simulink model "MotionControl"  (R2015b)
settings: Solver=ode3  StartTime=0.0  StopTime=inf  FixedStep=0.05  RelTol=1e-3
undefined symbols (not defined in the file or in its folder): C_nuParams, D, D_nuParams, InitialPos, invM, invT, invThrustAloc, K2, K3, K4, Ki, MAPP1, MAPP2, MAPP3, Sat1Low, Sat1Up, Sat2Low, Sat2Up, Th1, Th2, Th3, Tr, wni, wniCeta2, wnisquared, X, Y, Z
libraries: robotlib x14, realtime_pacer_lib x1
settings Model: Creator=einar  LastModifiedBy=Einar Ueland
settings DataIOCC: ReturnWorkspaceOutputs=on
settings OptimizationCC: OptimizeModelRefInitCode=on  LifeSpan=Inf  MaxStackSize=64
settings DebuggingCC: ReadBeforeWriteMsg=DisableAll  WriteAfterWriteMsg=DisableAll  WriteAfterReadMsg=DisableAll  MultiTaskDSMMsg=none
settings HardwareCC: ProdBitPerPointer=32  ProdLargestAtomicFloat=None  ProdIntDivRoundTo=Undefined  ProdEndianess=Unspecified  ProdWordSize=32  ProdHWDeviceType=Generic->Unspecified (assume 32-bit Generic)
settings ModelReferenceCC: UpdateModelReferenceTargets=IfOutOfDate
settings SFSimCC: SFSimEcho=off
settings RTWCC: SystemTargetFile=ert.tlc  TemplateMakefile=ert_default_tmf  Description=Embedded Coder  Toolchain=Catkin  TargetLang=C++
settings CodeAppCC: IgnoreCustomStorageClasses=off
settings ERTTargetCC: SupportContinuousTime=on

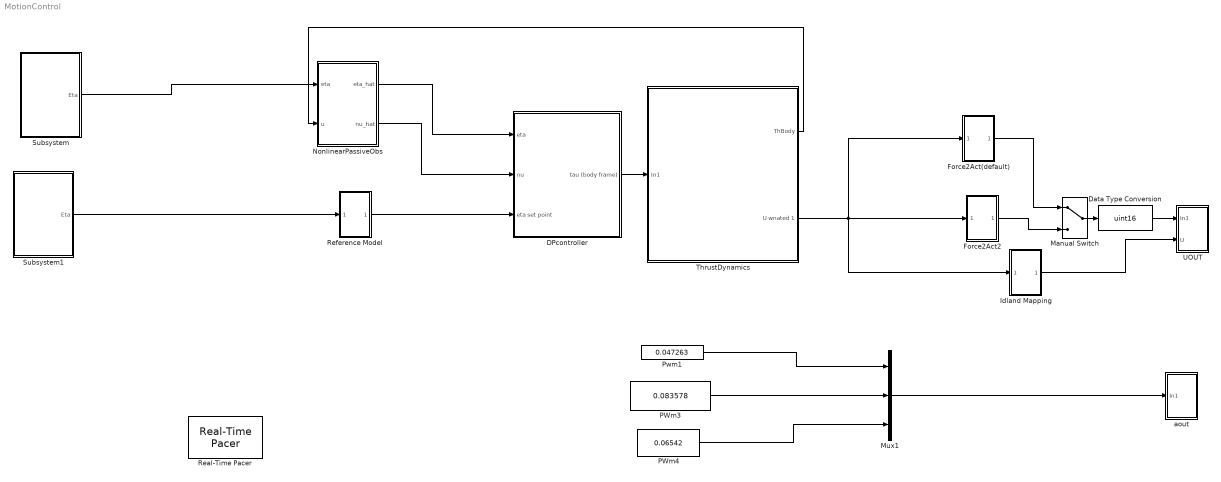
== system MotionControl ==
  DPcontroller : Subsystem
  Data Type Conversion : DataTypeConversion  OutDataTypeStr=uint16
  Force2Act(default) : Subsystem
  Force2Act2 : Subsystem
  Idland Mapping : Subsystem
  Manual Switch : ManualSwitch
  Mux1 : Mux  Inputs=3
  NonlinearPassiveObs : Subsystem
  PWm3 : Constant  Value=0.083578
  PWm4 : Constant  Value=0.06542
  Pwm1 : Constant  Value=0.047263
  Real-Time Pacer : realtime_pacer_lib/Real-Time Pacer  simTimePerRealTime=1
  Reference Model : Subsystem
  Subsystem : Subsystem
  Subsystem1 : Subsystem
  ThrustDynamics : Subsystem
  UOUT : Subsystem
  aout : Subsystem
  wires:
  NonlinearPassiveObs/2(nu_hat) -> DPcontroller/2(nu)
  DPcontroller/1(tau (body frame)) -> ThrustDynamics/1(In1)
  ThrustDynamics/1("ThBody ") -> NonlinearPassiveObs/2(u)
  Reference Model/1(Out1) -> DPcontroller/3(eta set point)
  Subsystem/1(Eta) -> NonlinearPassiveObs/1(eta)
  Subsystem1/1(Eta) -> Reference Model/1(In1)
  Force2Act2/1(Out1) -> Manual Switch/2
  Pwm1/1 -> Mux1/1
  PWm3/1 -> Mux1/2
  PWm4/1 -> Mux1/3
  Mux1/1 -> aout/1(In1)
  NonlinearPassiveObs/1(eta_hat) -> DPcontroller/1(eta)
  ThrustDynamics/2(U wnated 1) -> Force2Act(default)/1(In1), Force2Act2/1(In1), Idland Mapping/1(In1)
  Data Type Conversion/1 -> UOUT/1(In1)
  Idland Mapping/1(Out1) -> UOUT/2(U)
  Manual Switch/1 -> Data Type Conversion/1
  Force2Act(default)/1(Out1) -> Manual Switch/1

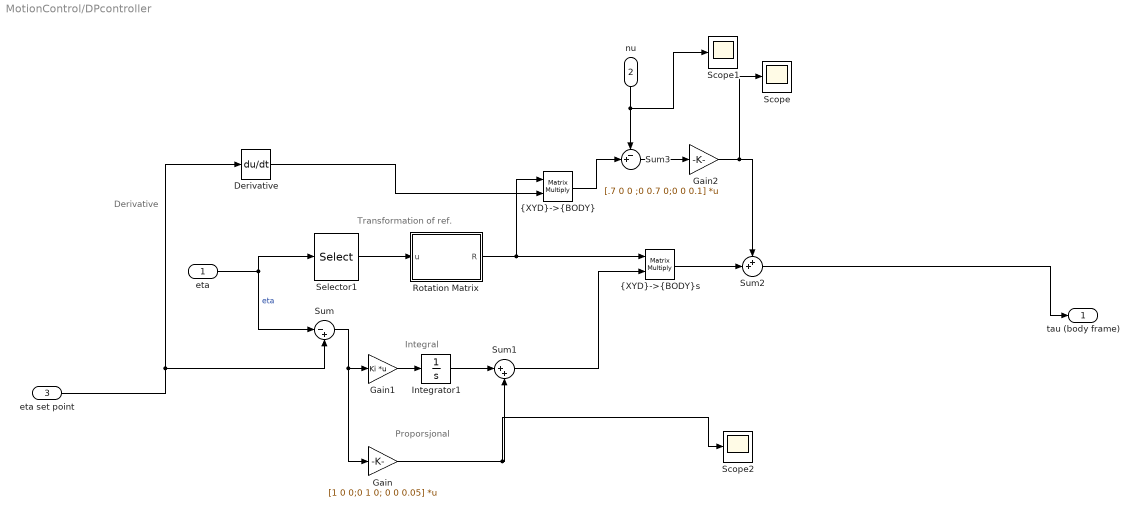
== system MotionControl/DPcontroller ==
  note: Integral
  note: Proporsjonal
  note: Transformation of ref.
  note: Derivative
  eta : Inport
  nu : Inport  Port=2
  eta set point : Inport  Port=3
  Derivative : Derivative
  Gain : Gain  Gain=[1 0 0;0 1 0; 0 0 0.05]  Multiplication=Matrix(K*u)
  Gain1 : Gain  Gain=Ki  Multiplication=Matrix(K*u)
  Gain2 : Gain  Gain=[.7 0 0 ;0 0.7 0;0 0 0.1]  Multiplication=Matrix(K*u)
  Integrator1 : Integrator  InitialCondition=[0;0;0]  LimitOutput=on  UpperSaturationLimit=[1;1;1]  LowerSaturationLimit=[-1;-1;-1]
  Rotation Matrix : MATLAB Function  TreatAsAtomicUnit=on
  Scope : Scope
  Scope1 : Scope
  Scope2 : Scope
  Selector1 : Selector  InputPortWidth=3  IndexOptions=Index vector (dialog)  Indices=[3]  OutputSizes=1
  Sum : Sum  Inputs=|-+
  Sum1 : Sum  Inputs=|++
  Sum2 : Sum  Inputs=++|
  Sum3 : Sum  Inputs=-+|
  "{XYD}->{BODY}" : Product  Multiplication=Matrix(*)
  "{XYD}->{BODY}s" : Product  Multiplication=Matrix(*)
  tau (body frame) : Outport
  wires:
  eta/1 -> Selector1/1, Sum/1  "eta"
  Sum/1 -> Gain1/1, Gain/1
  Selector1/1 -> Rotation Matrix/1(u)
  Rotation Matrix/1(R) -> "{XYD}->{BODY}"/1, "{XYD}->{BODY}s"/1
  Sum2/1 -> tau (body frame)/1
  Gain1/1 -> Integrator1/1
  Gain/1 -> Scope2/1, Sum1/2
  Sum1/1 -> "{XYD}->{BODY}s"/2
  Derivative/1 -> "{XYD}->{BODY}"/2
  "{XYD}->{BODY}s"/1 -> Sum2/2
  nu/1 -> Scope1/1, Sum3/1
  "{XYD}->{BODY}"/1 -> Sum3/2
  Sum3/1 -> Gain2/1
  Gain2/1 -> Scope/1, Sum2/1
  eta set point/1 -> Sum/2, Derivative/1
  Integrator1/1 -> Sum1/1

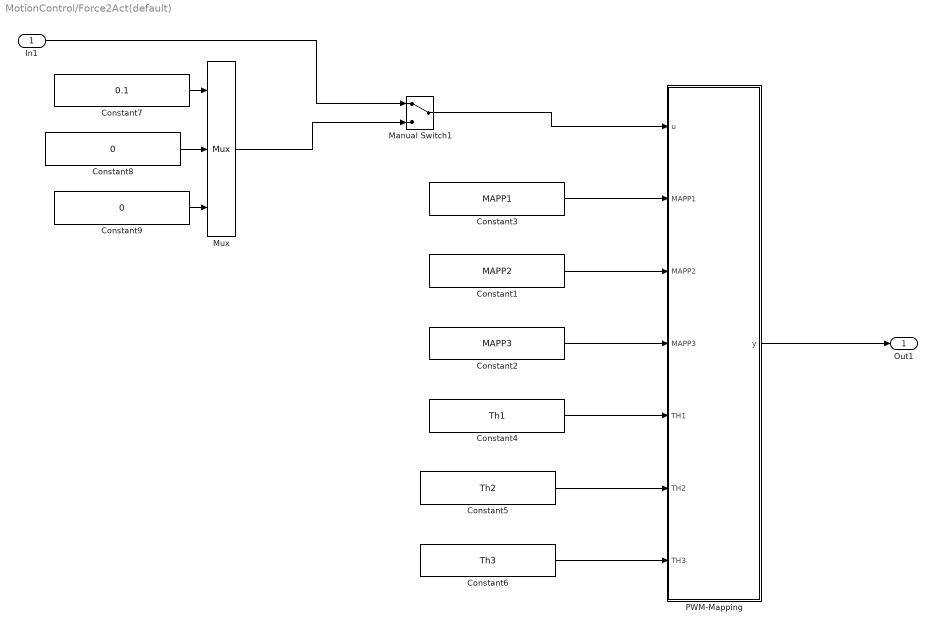
== system MotionControl/Force2Act(default) ==
  In1 : Inport
  Constant1 : Constant  Value=MAPP2
  Constant2 : Constant  Value=MAPP3
  Constant3 : Constant  Value=MAPP1
  Constant4 : Constant  Value=Th1
  Constant5 : Constant  Value=Th2
  Constant6 : Constant  Value=Th3
  Constant7 : Constant  Value=0.1
  Constant8 : Constant  Value=0
  Constant9 : Constant  Value=0
  Manual Switch1 : ManualSwitch
  Mux : Mux  Inputs=3
  PWM-Mapping : MATLAB Function  TreatAsAtomicUnit=on
  Out1 : Outport
  wires:
  Manual Switch1/1 -> PWM-Mapping/1(u)
  Constant4/1 -> PWM-Mapping/5(TH1)
  Constant6/1 -> PWM-Mapping/7(TH3)
  Constant5/1 -> PWM-Mapping/6(TH2)
  Constant3/1 -> PWM-Mapping/2(MAPP1)
  Constant1/1 -> PWM-Mapping/3(MAPP2)
  Constant2/1 -> PWM-Mapping/4(MAPP3)
  PWM-Mapping/1(y) -> Out1/1
  In1/1 -> Manual Switch1/1
  Constant7/1 -> Mux/1
  Constant8/1 -> Mux/2
  Mux/1 -> Manual Switch1/2
  Constant9/1 -> Mux/3

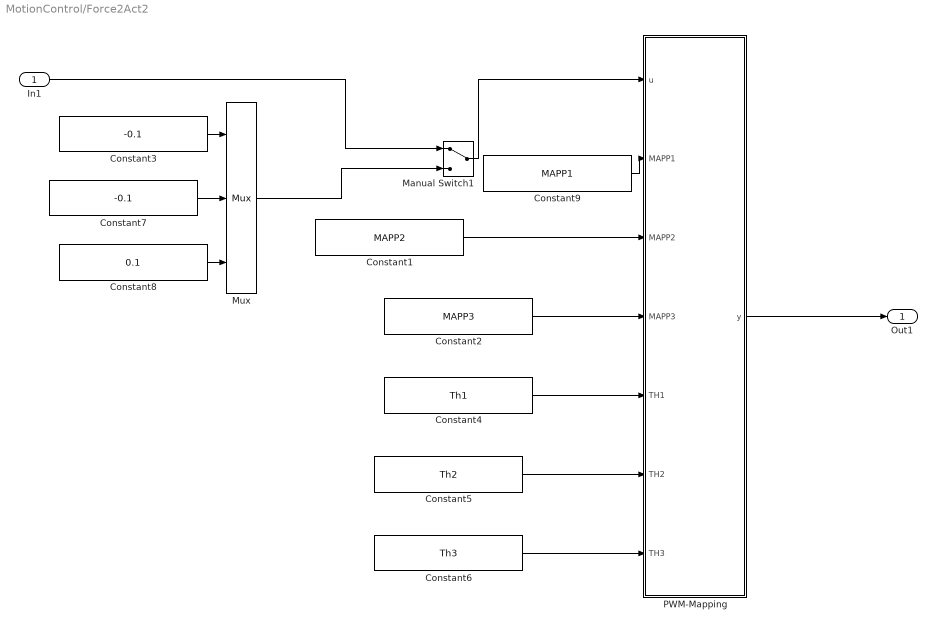
== system MotionControl/Force2Act2 ==
  In1 : Inport
  Constant1 : Constant  Value=MAPP2
  Constant2 : Constant  Value=MAPP3
  Constant3 : Constant  Value=-0.1
  Constant4 : Constant  Value=Th1
  Constant5 : Constant  Value=Th2
  Constant6 : Constant  Value=Th3
  Constant7 : Constant  Value=-0.1
  Constant8 : Constant  Value=0.1
  Constant9 : Constant  Value=MAPP1
  Manual Switch1 : ManualSwitch
  Mux : Mux  Inputs=3
  PWM-Mapping : MATLAB Function  TreatAsAtomicUnit=on
  Out1 : Outport
  wires:
  PWM-Mapping/1(y) -> Out1/1
  Constant2/1 -> PWM-Mapping/4(MAPP3)
  Constant1/1 -> PWM-Mapping/3(MAPP2)
  Manual Switch1/1 -> PWM-Mapping/1(u)
  Constant5/1 -> PWM-Mapping/6(TH2)
  Constant6/1 -> PWM-Mapping/7(TH3)
  Constant4/1 -> PWM-Mapping/5(TH1)
  In1/1 -> Manual Switch1/1
  Constant8/1 -> Mux/3
  Constant3/1 -> Mux/1
  Constant7/1 -> Mux/2
  Mux/1 -> Manual Switch1/2
  Constant9/1 -> PWM-Mapping/2(MAPP1)

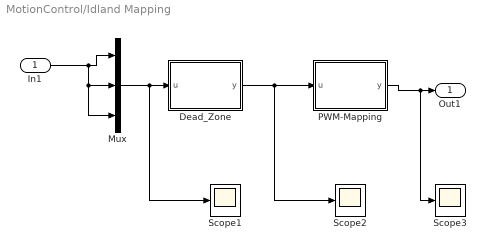
== system MotionControl/Idland Mapping ==
  In1 : Inport
  Dead_Zone : MATLAB Function  TreatAsAtomicUnit=on
  Mux : Mux  Inputs=3
  PWM-Mapping : MATLAB Function  TreatAsAtomicUnit=on
  Scope1 : Scope
  Scope2 : Scope
  Scope3 : Scope
  Out1 : Outport
  wires:
  PWM-Mapping/1(y) -> Out1/1, Scope3/1
  Mux/1 -> Dead_Zone/1(u), Scope1/1
  In1/1 -> Mux/3, Mux/2, Mux/1
  Dead_Zone/1(y) -> PWM-Mapping/1(u), Scope2/1

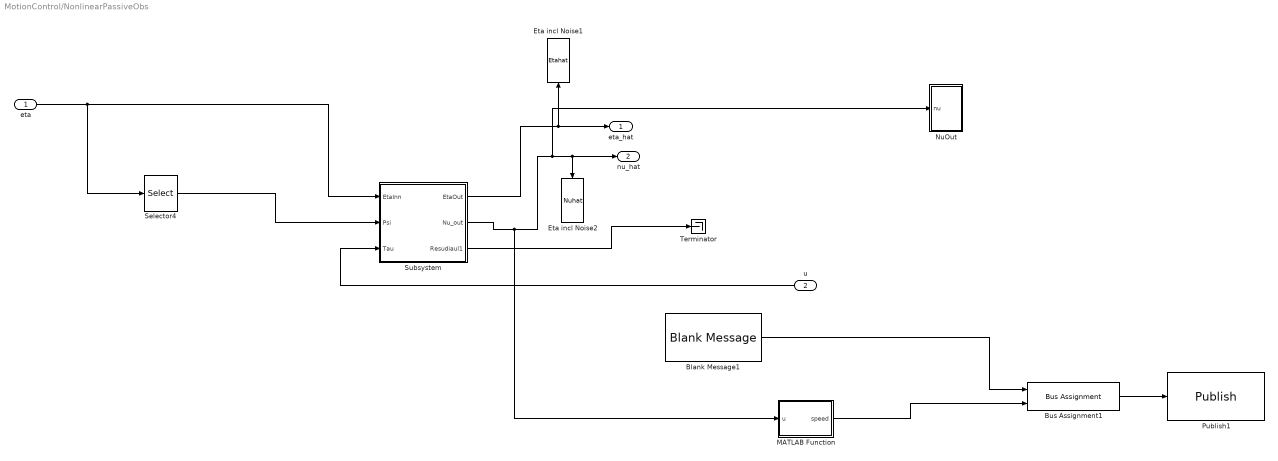
== system MotionControl/NonlinearPassiveObs ==
  eta : Inport
  u : Inport  Port=2
  Blank Message1 : robotlib/Blank Message  SourceLibraryInfo=This block requires Robotics System Toolbox  messageType=std_msgs/Float64  SampleTime=inf
  Bus Assignment1 : BusAssignment  AssignedSignals=Data
  Eta incl Noise1 : ToWorkspace  VariableName=Etahat  SaveFormat=Timeseries  SampleTime=-1
  Eta incl Noise2 : ToWorkspace  VariableName=Nuhat  SaveFormat=Timeseries  SampleTime=-1
  MATLAB Function : MATLAB Function  TreatAsAtomicUnit=on
  NuOut : Subsystem
  Publish1 : robotlib/Publish  SourceLibraryInfo=This block requires Robotics System Toolbox  topicSource=Specify your own  topic=/VesselSpeed  messageType=std_msgs/Float64  messageQueueLength=1
  Selector4 : Selector  InputPortWidth=3  IndexOptions=Index vector (dialog)  Indices=3  OutputSizes=1
  Subsystem : Subsystem
  Terminator : Terminator
  eta_hat : Outport
  nu_hat : Outport  Port=2
  wires:
  Subsystem/3("Resudiaul1 ") -> Terminator/1
  eta/1 -> Selector4/1, Subsystem/1(EtaInn)
  Selector4/1 -> Subsystem/2(Psi)
  u/1 -> Subsystem/3("Tau ")
  Subsystem/1("EtaOut ") -> Eta incl Noise1/1, eta_hat/1
  Bus Assignment1/1 -> Publish1/1
  Blank Message1/1 -> Bus Assignment1/1
  Subsystem/2("Nu_out ") -> MATLAB Function/1(u), NuOut/1("nu "), Eta incl Noise2/1, nu_hat/1
  MATLAB Function/1(speed) -> Bus Assignment1/2

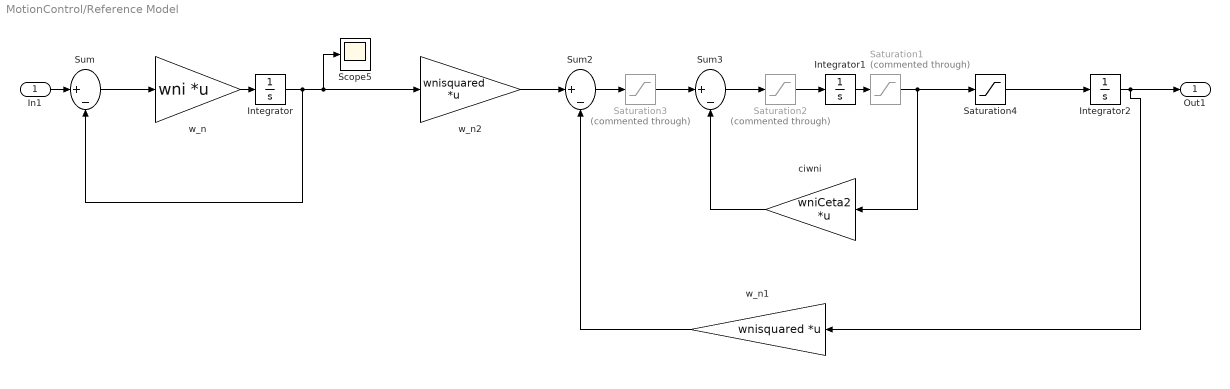
== system MotionControl/Reference Model ==
  In1 : Inport
  Integrator : Integrator  InitialCondition=[0;0;0]
  Integrator1 : Integrator  InitialCondition=[0 ;0; 0]
  Integrator2 : Integrator  InitialCondition=[0;0;0]
  Saturation1 : Saturate  Commented=through  UpperLimit=Sat2Up  LowerLimit=Sat2Low
  Saturation2 : Saturate  Commented=through  UpperLimit=Sat1Up  LowerLimit=Sat1Low
  Saturation3 : Saturate  Commented=through  UpperLimit=Sat1Up  LowerLimit=Sat1Low
  Saturation4 : Saturate  UpperLimit=Sat2Up  LowerLimit=Sat2Low
  Scope5 : Scope
  Sum : Sum  Inputs=|+-
  Sum2 : Sum  Inputs=|+-
  Sum3 : Sum  Inputs=|+-
  ciwni : Gain  Gain=wniCeta2  Multiplication=Matrix(K*u)
  w_n : Gain  Gain=wni  Multiplication=Matrix(K*u)
  w_n1 : Gain  Gain=wnisquared  Multiplication=Matrix(K*u)
  w_n2 : Gain  Gain=wnisquared  Multiplication=Matrix(K*u)
  Out1 : Outport
  wires:
  w_n/1 -> Integrator/1
  w_n2/1 -> Sum2/1
  Integrator/1 -> Scope5/1, w_n2/1, Sum/2
  Integrator2/1 -> Out1/1, w_n1/1
  ciwni/1 -> Sum3/2
  Saturation1/1 -> ciwni/1, Saturation4/1
  Saturation2/1 -> Integrator1/1
  Sum2/1 -> Saturation3/1
  Sum3/1 -> Saturation2/1
  Sum/1 -> w_n/1
  In1/1 -> Sum/1
  Integrator1/1 -> Saturation1/1
  w_n1/1 -> Sum2/2
  Saturation3/1 -> Sum3/1
  Saturation4/1 -> Integrator2/1

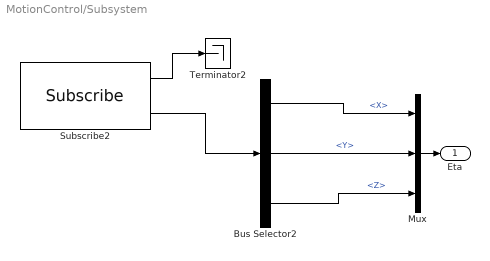
== system MotionControl/Subsystem ==
  Bus Selector2 : BusSelector  OutputSignals=X,Y,Z
  Mux : Mux  Inputs=3
  Subscribe2 : robotlib/Subscribe  SourceLibraryInfo=This block requires Robotics System Toolbox  topicSource=Specify your own  topic=/Eta  messageType=geometry_msgs/Vector3  sampleTime=-1  messageQueueLength=1
  Terminator2 : Terminator
  Eta : Outport
  wires:
  Bus Selector2/1 -> Mux/1  "<X>"
  Subscribe2/2 -> Bus Selector2/1
  Mux/1 -> Eta/1
  Subscribe2/1 -> Terminator2/1
  Bus Selector2/2 -> Mux/2  "<Y>"
  Bus Selector2/3 -> Mux/3  "<Z>"

== system MotionControl/Subsystem1 ==
  Bus Selector2 : BusSelector  OutputSignals=X,Y,Z
  Mux : Mux  Inputs=3
  Subscribe2 : robotlib/Subscribe  SourceLibraryInfo=This block requires Robotics System Toolbox  topicSource=Specify your own  topic=/Position  messageType=geometry_msgs/Vector3  sampleTime=-1  messageQueueLength=1
  Terminator2 : Terminator
  Eta : Outport
  wires:
  Subscribe2/2 -> Bus Selector2/1
  Mux/1 -> Eta/1
  Subscribe2/1 -> Terminator2/1
  Bus Selector2/1 -> Mux/1  "<X>"
  Bus Selector2/2 -> Mux/2  "<Y>"
  Bus Selector2/3 -> Mux/3  "<Z>"

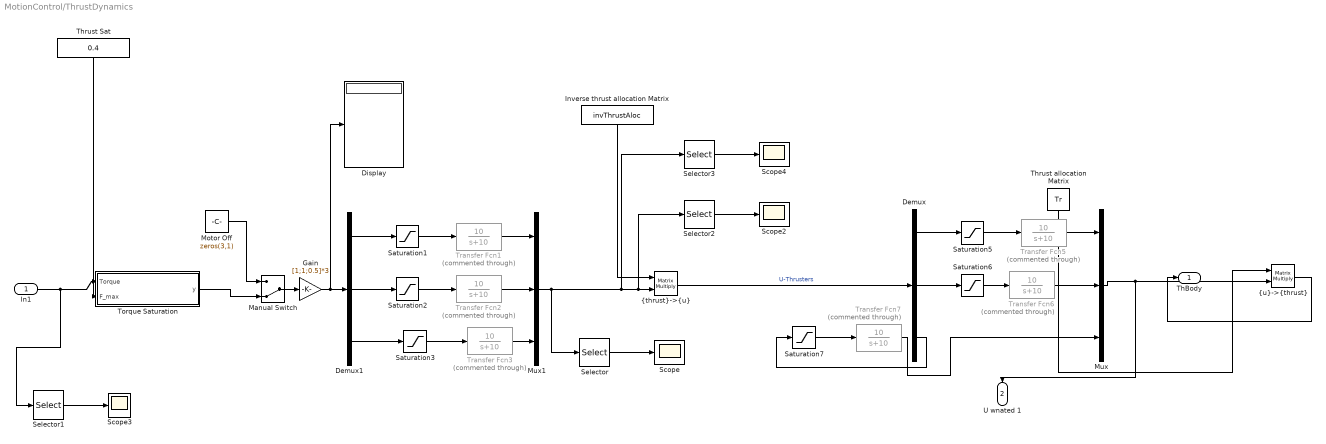
== system MotionControl/ThrustDynamics ==
  In1 : Inport
  Demux : Demux  Outputs=3
  Demux1 : Demux  Outputs=3
  Display : Display
  Gain : Gain  Gain=[1;1;0.5]*3
  Inverse thrust allocation Matrix : Constant  Value=invThrustAloc
  Manual Switch : ManualSwitch  CurrentSetting=0
  Motor Off : Constant  Value=zeros(3,1)
  Mux : Mux  Inputs=3
  Mux1 : Mux  Inputs=3
  Saturation1 : Saturate  UpperLimit=1  LowerLimit=-1  ZeroCross=off
  Saturation2 : Saturate  UpperLimit=1  LowerLimit=-1  ZeroCross=off
  Saturation3 : Saturate  UpperLimit=0.05  LowerLimit=-0.05  ZeroCross=off
  Saturation5 : Saturate  UpperLimit=4  LowerLimit=-4  ZeroCross=off
  Saturation6 : Saturate  UpperLimit=4  LowerLimit=-4  ZeroCross=off
  Saturation7 : Saturate  UpperLimit=4  LowerLimit=-4  ZeroCross=off
  Scope{,2..4} (4 alike) : Scope
  Selector : Selector  InputPortWidth=3  IndexOptions=Index vector (dialog)  Indices=[3]  OutputSizes=1
  Selector1 : Selector  InputPortWidth=3  IndexOptions=Index vector (dialog)  Indices=[3]  OutputSizes=1
  Selector2 : Selector  InputPortWidth=3  IndexOptions=Index vector (dialog)  Indices=2  OutputSizes=1
  Selector3 : Selector  InputPortWidth=3  IndexOptions=Index vector (dialog)  Indices=1  OutputSizes=1
  Thrust Sat : Constant  Value=0.4
  Thrust allocation Matrix : Constant  Value=Tr
  Torque Saturation : MATLAB Function  TreatAsAtomicUnit=on
  Transfer Fcn{1..3,5..7} (6 alike) : TransferFcn  Commented=through  Numerator=[10]  Denominator=[1 10]
  "{thrust}->{u}" : Product  Multiplication=Matrix(*)
  "{u}->{thrust}" : Product  Multiplication=Matrix(*)
  "ThBody " : Outport
  U wnated 1 : Outport  Port=2
  wires:
  Demux/1 -> Saturation5/1
  Demux/2 -> Saturation6/1
  Demux/3 -> Saturation7/1
  "{u}->{thrust}"/1 -> "ThBody "/1
  Thrust allocation Matrix/1 -> "{u}->{thrust}"/1
  Mux/1 -> "{u}->{thrust}"/2, U wnated 1/1
  "{thrust}->{u}"/1 -> Demux/1  "U-Thrusters"
  Inverse thrust allocation Matrix/1 -> "{thrust}->{u}"/1
  Saturation7/1 -> Transfer Fcn7/1
  Saturation6/1 -> Transfer Fcn6/1
  Saturation5/1 -> Transfer Fcn5/1
  Transfer Fcn5/1 -> Mux/1
  Transfer Fcn7/1 -> Mux/3
  Transfer Fcn6/1 -> Mux/2
  Selector/1 -> Scope/1
  In1/1 -> Selector1/1, Torque Saturation/1(Torque)
  Selector1/1 -> Scope3/1
  Demux1/1 -> Saturation1/1
  Demux1/2 -> Saturation2/1
  Demux1/3 -> Saturation3/1
  Saturation3/1 -> Transfer Fcn3/1
  Saturation2/1 -> Transfer Fcn2/1
  Saturation1/1 -> Transfer Fcn1/1
  Transfer Fcn1/1 -> Mux1/1
  Transfer Fcn3/1 -> Mux1/3
  Transfer Fcn2/1 -> Mux1/2
  Gain/1 -> Display/1, Demux1/1
  Mux1/1 -> Selector/1, Selector3/1, Selector2/1, "{thrust}->{u}"/2
  Selector2/1 -> Scope2/1
  Selector3/1 -> Scope4/1
  Thrust Sat/1 -> Torque Saturation/2(F_max)
  Torque Saturation/1(y) -> Manual Switch/2
  Manual Switch/1 -> Gain/1
  Motor Off/1 -> Manual Switch/1

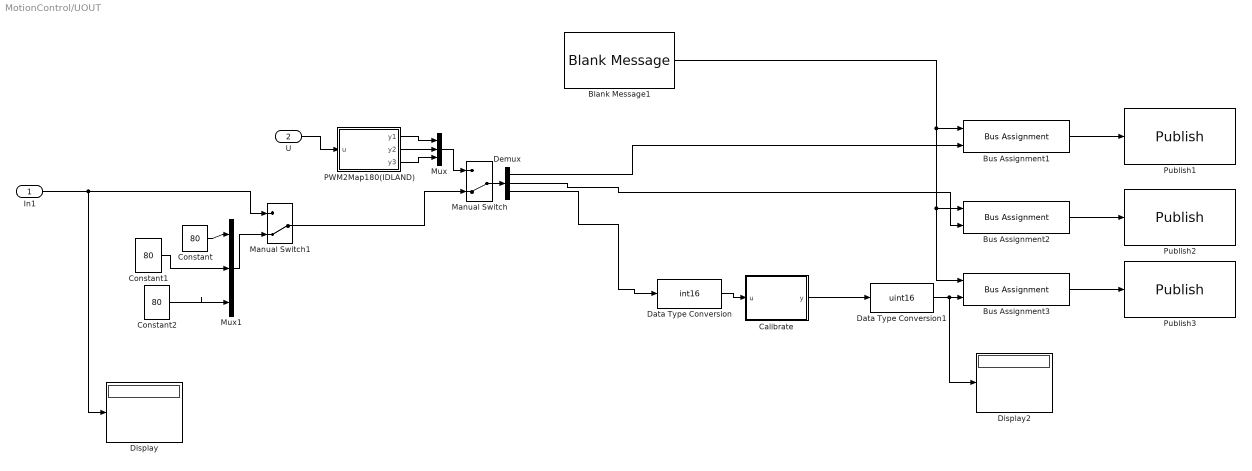
== system MotionControl/UOUT ==
  In1 : Inport
  U : Inport  Port=2
  Blank Message1 : robotlib/Blank Message  SourceLibraryInfo=This block requires Robotics System Toolbox  messageType=std_msgs/UInt16  SampleTime=inf
  Bus Assignment1 : BusAssignment  AssignedSignals=Data
  Bus Assignment2 : BusAssignment  AssignedSignals=Data
  Bus Assignment3 : BusAssignment  AssignedSignals=Data
  Calibrate : MATLAB Function  TreatAsAtomicUnit=on
  Constant : Constant  Value=80  OutDataTypeStr=uint16
  Constant1 : Constant  Value=80  OutDataTypeStr=uint16
  Constant2 : Constant  Value=80  OutDataTypeStr=uint16
  Data Type Conversion : DataTypeConversion  OutDataTypeStr=int16
  Data Type Conversion1 : DataTypeConversion  OutDataTypeStr=uint16
  Demux : Demux  Outputs=3
  Display : Display
  Display2 : Display
  Manual Switch : ManualSwitch  CurrentSetting=0
  Manual Switch1 : ManualSwitch  CurrentSetting=0
  Mux : Mux  Inputs=3
  Mux1 : Mux  Inputs=3
  "PWM2Map180(IDLAND) " : MATLAB Function  TreatAsAtomicUnit=on
  Publish1 : robotlib/Publish  SourceLibraryInfo=This block requires Robotics System Toolbox  topicSource=Specify your own  topic=/Thrust1  messageType=std_msgs/UInt16  messageQueueLength=1
  Publish2 : robotlib/Publish  SourceLibraryInfo=This block requires Robotics System Toolbox  topicSource=Specify your own  topic=/Thrust2  messageType=std_msgs/UInt16  messageQueueLength=1
  Publish3 : robotlib/Publish  SourceLibraryInfo=This block requires Robotics System Toolbox  topicSource=Specify your own  topic=/Thrust3  messageType=std_msgs/UInt16  messageQueueLength=1
  wires:
  Bus Assignment3/1 -> Publish3/1
  Demux/2 -> Bus Assignment2/2
  Bus Assignment1/1 -> Publish1/1
  Blank Message1/1 -> Bus Assignment3/1, Bus Assignment2/1, Bus Assignment1/1
  In1/1 -> Manual Switch1/1, Display/1
  Demux/1 -> Bus Assignment1/2
  Bus Assignment2/1 -> Publish2/1
  U/1 -> "PWM2Map180(IDLAND) "/1(u)
  "PWM2Map180(IDLAND) "/2(y2) -> Mux/2
  "PWM2Map180(IDLAND) "/3(y3) -> Mux/3
  "PWM2Map180(IDLAND) "/1(y1) -> Mux/1
  Mux/1 -> Manual Switch/1
  Manual Switch/1 -> Demux/1
  Mux1/1 -> Manual Switch1/2
  Constant/1 -> Mux1/1
  Constant1/1 -> Mux1/2
  Constant2/1 -> Mux1/3
  Manual Switch1/1 -> Manual Switch/2
  Demux/3 -> Data Type Conversion/1
  Data Type Conversion/1 -> Calibrate/1(u)
  Data Type Conversion1/1 -> Display2/1, Bus Assignment3/2
  Calibrate/1(y) -> Data Type Conversion1/1

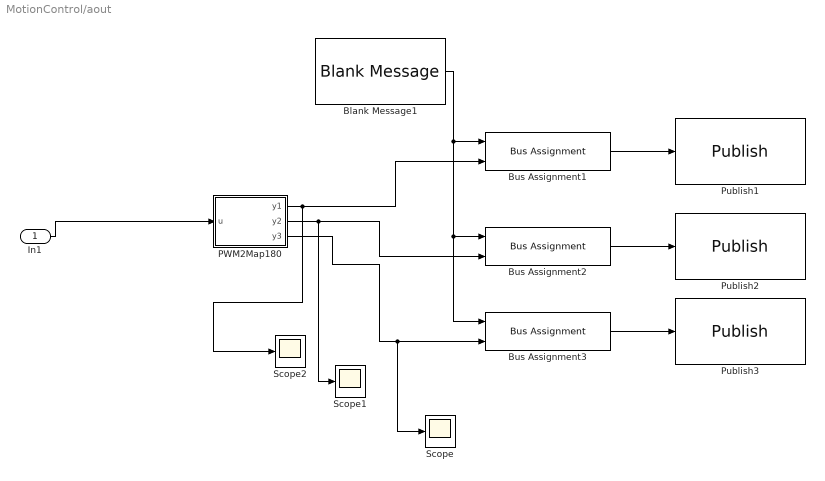
== system MotionControl/aout ==
  In1 : Inport
  Blank Message1 : robotlib/Blank Message  SourceLibraryInfo=This block requires Robotics System Toolbox  messageType=std_msgs/UInt16  SampleTime=inf
  Bus Assignment1 : BusAssignment  AssignedSignals=Data
  Bus Assignment2 : BusAssignment  AssignedSignals=Data
  Bus Assignment3 : BusAssignment  AssignedSignals=Data
  "PWM2Map180 " : MATLAB Function  TreatAsAtomicUnit=on
  Publish1 : robotlib/Publish  SourceLibraryInfo=This block requires Robotics System Toolbox  topicSource=Specify your own  topic=/a1  messageType=std_msgs/UInt16  messageQueueLength=1
  Publish2 : robotlib/Publish  SourceLibraryInfo=This block requires Robotics System Toolbox  topicSource=Specify your own  topic=/a2  messageType=std_msgs/UInt16  messageQueueLength=1
  Publish3 : robotlib/Publish  SourceLibraryInfo=This block requires Robotics System Toolbox  topicSource=Specify your own  topic=/a3  messageType=std_msgs/UInt16  messageQueueLength=1
  Scope : Scope
  Scope1 : Scope
  Scope2 : Scope
  wires:
  Bus Assignment2/1 -> Publish2/1
  "PWM2Map180 "/1(y1) -> Bus Assignment1/2, Scope2/1
  "PWM2Map180 "/3(y3) -> Bus Assignment3/2, Scope/1
  In1/1 -> "PWM2Map180 "/1(u)
  Blank Message1/1 -> Bus Assignment1/1, Bus Assignment2/1, Bus Assignment3/1
  Bus Assignment1/1 -> Publish1/1
  "PWM2Map180 "/2(y2) -> Scope1/1, Bus Assignment2/2
  Bus Assignment3/1 -> Publish3/1

== system MotionControl/NonlinearPassiveObs/NuOut ==
  "nu " : Inport
  Blank Message1 : robotlib/Blank Message  SourceLibraryInfo=This block requires Robotics System Toolbox  messageType=geometry_msgs/Vector3  SampleTime=inf
  Bus Assignment3 : BusAssignment  AssignedSignals=X,Y,Z
  Demux : Demux  Outputs=3
  Publish3 : robotlib/Publish  SourceLibraryInfo=This block requires Robotics System Toolbox  topicSource=Specify your own  topic=/nu  messageType=geometry_msgs/Vector3  messageQueueLength=1
  wires:
  Bus Assignment3/1 -> Publish3/1
  Blank Message1/1 -> Bus Assignment3/1
  "nu "/1 -> Demux/1
  Demux/1 -> Bus Assignment3/2
  Demux/2 -> Bus Assignment3/3
  Demux/3 -> Bus Assignment3/4

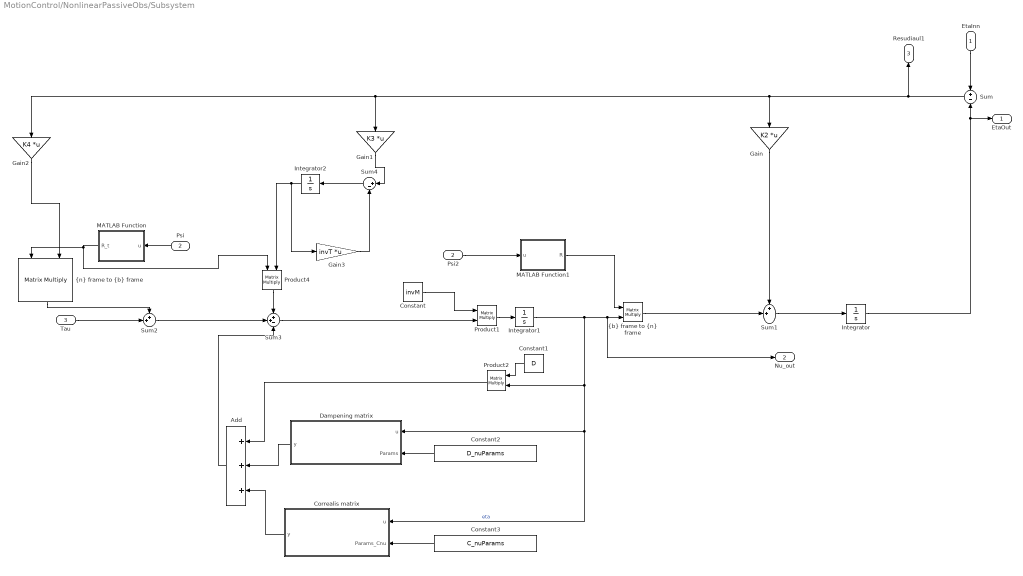
== system MotionControl/NonlinearPassiveObs/Subsystem ==
  EtaInn : Inport
  Psi : Inport  Port=2
  "Tau " : Inport  Port=3
  Add : Sum  Inputs=+++
  Constant : Constant  Value=invM
  Constant1 : Constant  Value=D
  Constant2 : Constant  Value=D_nuParams
  Constant3 : Constant  Value=C_nuParams
  Correalis matrix : MATLAB Function  TreatAsAtomicUnit=on
  Dampening matrix : MATLAB Function  TreatAsAtomicUnit=on
  Gain : Gain  Gain=K2  Multiplication=Matrix(K*u)
  Gain1 : Gain  Gain=K3  Multiplication=Matrix(K*u)
  Gain2 : Gain  Gain=K4  Multiplication=Matrix(K*u)
  Gain3 : Gain  Gain=invT  Multiplication=Matrix(K*u)
  Integrator : Integrator  InitialCondition=InitialPos
  Integrator1 : Integrator
  Integrator2 : Integrator  InitialCondition=[0;0;0]
  MATLAB Function : MATLAB Function  TreatAsAtomicUnit=on
  MATLAB Function1 : MATLAB Function  TreatAsAtomicUnit=on
  Product1 : Product  Multiplication=Matrix(*)
  Product2 : Product  Multiplication=Matrix(*)
  Product4 : Product  Multiplication=Matrix(*)
  Psi2 : InportShadow  Port=2
  Sum : Sum  Inputs=+|-
  Sum1 : Sum  Inputs=++|
  Sum2 : Sum  Inputs=++|
  Sum3 : Sum  Inputs=++-
  Sum4 : Sum  Inputs=|+-
  "{b} frame to {n} frame" : Product  Multiplication=Matrix(*)
  "{n} frame to {b} frame" : Product  Multiplication=Matrix(*)
  "EtaOut " : Outport
  "Nu_out " : Outport  Port=2
  "Resudiaul1 " : Outport  Port=3
  wires:
  Add/1 -> Sum3/3
  Correalis matrix/1(y) -> Add/3
  Dampening matrix/1(y) -> Add/2
  Product2/1 -> Add/1
  Integrator1/1 -> Product2/2, Dampening matrix/1(u), Correalis matrix/1(u), "Nu_out "/1, "{b} frame to {n} frame"/2  "eta"
  Constant3/1 -> Correalis matrix/2(Params_Cnu)
  Constant2/1 -> Dampening matrix/2(Params)
  Gain2/1 -> "{n} frame to {b} frame"/2
  EtaInn/1 -> Sum/1
  Sum/1 -> "Resudiaul1 "/1, Gain2/1, Gain1/1, Gain/1
  Gain/1 -> Sum1/1
  Sum1/1 -> Integrator/1
  Integrator/1 -> Sum/2, "EtaOut "/1
  Psi/1 -> MATLAB Function/1(u)
  "{n} frame to {b} frame"/1 -> Sum2/1
  "Tau "/1 -> Sum2/2
  Constant/1 -> Product1/1
  Product1/1 -> Integrator1/1
  Constant1/1 -> Product2/1
  Sum2/1 -> Sum3/2
  Sum3/1 -> Product1/2
  Psi2/1 -> MATLAB Function1/1(u)
  MATLAB Function1/1(R) -> "{b} frame to {n} frame"/1
  MATLAB Function/1(R_t) -> Product4/1, "{n} frame to {b} frame"/1
  "{b} frame to {n} frame"/1 -> Sum1/2
  Gain1/1 -> Sum4/1
  Sum4/1 -> Integrator2/1
  Integrator2/1 -> Product4/2, Gain3/1
  Gain3/1 -> Sum4/2
  Product4/1 -> Sum3/1

== matlab function MotionControl/DPcontroller/Rotation Matrix ==
  data: u input; R output
function R = fcn(u)
RotPhi=[cos(u) -sin(u) 0;sin(u) cos(u) 0 ;0 0 1];
R = RotPhi';
%R=[RotPhi(1:2,:);[0 0 0;0 0 0;0 0 0];RotPhi(3,:)]
end

== matlab function MotionControl/UOUT/PWM2Map180(IDLAND)  ==
  data: u input; y1 output; y2 output; y3 output
function [y1,y2,y3] = fcn(u)
%#codegen
y1=uint16((u(1)-0.027)*180/0.093);
y2=uint16((u(2)-0.027)*180/0.093);
y3=uint16((u(3)-0.027)*180/0.093);

== matlab function MotionControl/NonlinearPassiveObs/Subsystem/Correalis matrix ==
  data: u input; y output; Params_Cnu input
function y = fcn(u,Params_Cnu)
%#codegen
C=[0 Params_Cnu(2,1)*u(3) 0;-Params_Cnu(1,2)*u(3) 0 0;0 0 0];
y=C*u;

== matlab function MotionControl/NonlinearPassiveObs/Subsystem/Dampening matrix ==
  data: u input; y output; Params input
function y = fcn(u,Params)
%#codegen
Dnu=[Params(1,1)*abs(u(1)) 0 0;0 Params(2,2)*abs(u(2)) 0;0 0 0];
y=Dnu*u;

== matlab function MotionControl/aout/PWM2Map180  ==
  data: u input; y1 output; y2 output; y3 output
function [y1,y2,y3] = fcn(u)
%#codegen
y1=uint16((u(1)-0.027)*180/0.093);
y2=uint16((u(2)-0.027)*180/0.093);
y3=uint16((u(3)-0.027)*180/0.093);

== matlab function MotionControl/Force2Act(default)/PWM-Mapping ==
  data: u input; y output; MAPP1 input; MAPP2 input; MAPP3 input; TH1 input; TH2 input; TH3 input
function y = fcn(u,MAPP1,MAPP2,MAPP3,TH1,TH2,TH3)
y=[0 ;0;0]
u(3)=-u(3);
MAPP3=-MAPP1;
TH3=TH1

if u(1)>max(MAPP1)
    u(1)=max(MAPP1)
elseif u(1)<min(MAPP1)
u(1)=min(MAPP1);
end

if u(2)>max(MAPP2)
    u(2)=max(MAPP2)
elseif u(2)<min(MAPP2)
u(2)=min(MAPP2);
end

if u(3)>max(MAPP3)
    u(3)=max(MAPP3)
elseif u(3)<min(MAPP3)
u(3)=min(MAPP3);
end

y(1)=interp1(MAPP1,TH1,u(1))
y(2)=interp1(MAPP2,TH2,u(2))
y(3)=interp1(MAPP3,TH3,u(3))

if abs(u(1))<0.01
    y(1)=80;
end
if abs(u(2))<0.01
    y(2)=80;
end
if abs(u(3))<0.01
    y(3)=80;
end

== matlab function MotionControl/Force2Act2/PWM-Mapping ==
  data: u input; y output; MAPP1 input; MAPP2 input; MAPP3 input; TH1 input; TH2 input; TH3 input
function y = fcn(u,MAPP1,MAPP2,MAPP3,TH1,TH2,TH3)
y=[0 ;0;0]
u(3)=-u(3);
if u(1)>max(MAPP1)
    u(1)=max(MAPP1)
elseif u(1)<min(MAPP1)
u(1)=min(MAPP1);
end

if u(2)>max(MAPP2)
    u(2)=max(MAPP2)
elseif u(2)<min(MAPP2)
u(2)=min(MAPP2);
end

if u(3)>max(MAPP3)
    u(3)=max(MAPP3)
elseif u(3)<min(MAPP3)
u(3)=min(MAPP3);
end

y(1)=interp1(MAPP1,TH1,u(1))
y(2)=interp1(MAPP2,TH2,u(2))
y(3)=interp1(MAPP3,TH3,u(3))

if abs(u(1))<0.01
    y(1)=80;
end
if abs(u(2))<0.01
    y(2)=80;
end
if abs(u(3))<0.01
    y(3)=80;
end

== matlab function MotionControl/Idland Mapping/Dead_Zone ==
  data: u input; y output
function y = fcn(u)
%#codegen
y=[0 ;0 ;0]
for i=1:3
if (u(i)<-0.005);
    y(i)=u(i)*0.8-0.15;
elseif (u(i)>0.005)
    y(i)=u(i)*0.8+0.15
end
end

== matlab function MotionControl/Idland Mapping/PWM-Mapping ==
  data: u input; y output
function y = fcn(u)
y=(u.*0.0255)+(0.0685)
end

== matlab function MotionControl/UOUT/Calibrate ==
  data: u input; y output
function y  = fcn(u)
y=u;
if u<80
y=y+3
end
%     y=y+1;
% elseif u<80
%     y=y+3;
% end

== matlab function MotionControl/NonlinearPassiveObs/Subsystem/MATLAB Function ==
  data: u input; R_t output
function R_t = fcn(u)
RotPhi=[cos(u) -sin(u) 0;sin(u) cos(u) 0 ;0 0 1];
R_t = RotPhi';
%R=[RotPhi(1:2,:);[0 0 0;0 0 0;0 0 0];RotPhi(3,:)]
end

== matlab function MotionControl/NonlinearPassiveObs/MATLAB Function ==
  data: u input; speed output
function speed = fcn(u)
%#codegen
speed=norm(u(1:2));

== matlab function MotionControl/NonlinearPassiveObs/Subsystem/MATLAB Function1 ==
  data: u input; R output
function R = fcn(u)
RotPhi=[cos(u) -sin(u) 0;sin(u) cos(u) 0 ;0 0 1];
R = RotPhi;
end

== matlab function MotionControl/ThrustDynamics/Torque Saturation ==
  data: Torque input; y output; F_max input
function y = fcn(Torque,F_max)
Com_Torque=norm(Torque(1:2));
if Com_Torque>F_max
Torque(1:2,1)=Torque(1:2,1).*(F_max/Com_Torque)    ;
end
T_max=0.3;
if abs(Torque(3))>T_max
Torque(3)=T_max*Torque(3)/abs(Torque(3));
end;
y=Torque;
